simulink model "gm_controller_only"  (R2025a)
settings: Solver=FixedStepDiscrete  StartTime=0.0  StopTime=0.2  FixedStep=5e-05  RelTol=1e-3
settings Model: Creator=Edith  LastModifiedBy=HP
settings OptimizationCC: BlockReduction=off  ConditionallyExecuteInputs=off  DefaultParameterBehavior=Inlined
settings DebuggingCC: AlgebraicLoopMsg=error  InheritedTsInSrcMsg=none
settings HardwareCC: ProdBitPerPointer=32.0  ProdBitPerSizeT=32.0  ProdBitPerPtrDiffT=32.0  ProdLargestAtomicFloat=None  ProdIntDivRoundTo=Undefined  ProdEndianess=Unspecified  ProdWordSize=32.0  ProdHWDeviceType=ASIC/FPGA->ASIC/FPGA  TargetBitPerPointer=64.0  TargetBitPerSizeT=64.0  TargetBitPerPtrDiffT=64.0  TargetLongLongMode=on  TargetIntDivRoundTo=Zero  TargetEndianess=LittleEndian  TargetWordSize=64.0  TargetHWDeviceType=Custom Processor->MATLAB Host Computer  ProdEqTarget=off

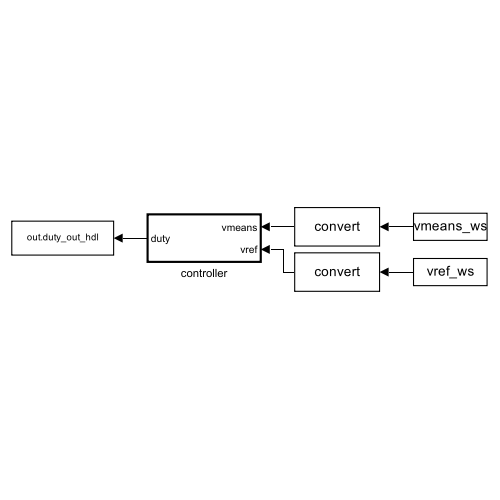
[thumbnail: Simulink's stored preview of the top-level diagram]
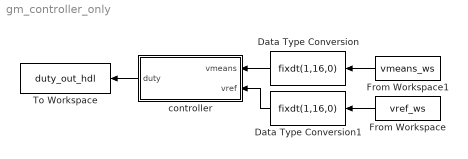
== system gm_controller_only ==
  Data Type Conversion : DataTypeConversion  OutDataTypeStr=fixdt(1,16,0)  SaturateOnIntegerOverflow=off  RndMeth=Floor
  Data Type Conversion1 : DataTypeConversion  OutDataTypeStr=fixdt(1,16,0)  SaturateOnIntegerOverflow=off  RndMeth=Floor
  From Workspace : FromWorkspace  VariableName=vref_ws
  From Workspace1 : FromWorkspace  VariableName=vmeans_ws
  To Workspace : ToWorkspace  VariableName=duty_out_hdl  SampleTime=-1
  controller : Subsystem  TreatAsAtomicUnit=on  SystemSampleTime=5e-5
  wires:
  From Workspace1/1 -> Data Type Conversion/1
  Data Type Conversion1/1 -> controller/2(vref)
  Data Type Conversion/1 -> controller/1(vmeans)
  From Workspace/1 -> Data Type Conversion1/1
  controller/1(duty) -> To Workspace/1

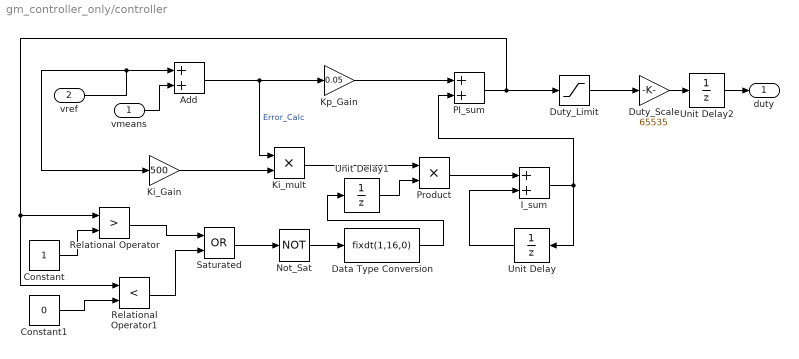
== system gm_controller_only/controller ==
  vmeans : Inport  OutDataTypeStr=fixdt(1,16,0)
  vref : Inport  Port=2
  Add : Sum  OutDataTypeStr=fixdt(1,16,0)  AccumDataTypeStr=fixdt(1,16,0)
  Constant : Constant  OutDataTypeStr=fixdt(1,16,0)  SampleTime=-1
  Constant1 : Constant  Value=0  OutDataTypeStr=fixdt(1,16,0)  SampleTime=-1
  Data Type Conversion : DataTypeConversion  OutDataTypeStr=fixdt(1,16,0)  SaturateOnIntegerOverflow=off  RndMeth=Floor
  Duty_Limit : Saturate  UpperLimit=1  LowerLimit=0  OutDataTypeStr=fixdt(1,16,0)
  Duty_Scale : Gain  Gain=65535  OutDataTypeStr=fixdt(1,16,0)
  I_sum : Sum  OutDataTypeStr=fixdt(1,16,0)  AccumDataTypeStr=fixdt(1,16,0)
  Ki_Gain : Gain  Gain=500  OutDataTypeStr=fixdt(1,16,0)
  Ki_mult : Product  OutDataTypeStr=fixdt(1,16,0)
  Kp_Gain : Gain  Gain=0.05  OutDataTypeStr=fixdt(1,16,0)
  Not_Sat : Logic  Operator=NOT  AllPortsSameDT=off  OutDataTypeStr=boolean
  PI_sum : Sum  OutDataTypeStr=fixdt(1,16,0)  AccumDataTypeStr=fixdt(1,16,0)
  Product : Product  OutDataTypeStr=fixdt(1,16,0)
  Relational Operator : RelationalOperator  Operator=>  OutDataTypeStr=boolean  RndMeth=Simplest  InputSameDT=off
  Relational Operator1 : RelationalOperator  Operator=<  OutDataTypeStr=boolean  RndMeth=Simplest  InputSameDT=off
  Saturated : Logic  Operator=OR  AllPortsSameDT=off  OutDataTypeStr=boolean
  Unit Delay : UnitDelay  SampleTime=5e-5  HasFrameUpgradeWarning=on
  Unit Delay1 : UnitDelay  SampleTime=5e-5  HasFrameUpgradeWarning=on
  Unit Delay2 : UnitDelay  SampleTime=5e-5  HasFrameUpgradeWarning=on
  duty : Outport
  wires:
  Unit Delay2/1 -> duty/1
  Duty_Scale/1 -> Unit Delay2/1
  Data Type Conversion/1 -> Unit Delay1/1
  Unit Delay1/1 -> Product/2
  Constant1/1 -> Relational Operator1/2
  Constant/1 -> Relational Operator/2
  Saturated/1 -> Not_Sat/1
  Relational Operator/1 -> Saturated/1
  Relational Operator1/1 -> Saturated/2
  I_sum/1 -> PI_sum/2, Unit Delay/1
  Duty_Limit/1 -> Duty_Scale/1
  Unit Delay/1 -> I_sum/2
  Ki_mult/1 -> Product/1
  Product/1 -> I_sum/1
  Not_Sat/1 -> Data Type Conversion/1
  PI_sum/1 -> Duty_Limit/1, Relational Operator/1, Relational Operator1/1
  Ki_Gain/1 -> Ki_mult/2
  Kp_Gain/1 -> PI_sum/1
  Add/1 -> Kp_Gain/1, Ki_mult/1  "Error_Calc"
  vmeans/1 -> Add/2
  vref/1 -> Add/1, Ki_Gain/1
